simulink model "battery_sim"  (R2022a)
settings: Solver=VariableStepAuto  StartTime=0.0  StopTime=10000  RelTol=1e-3
undefined symbols (not defined in the file): T_AMB
settings Model: Creator=Cristobal  LastModifiedBy=Cristobal

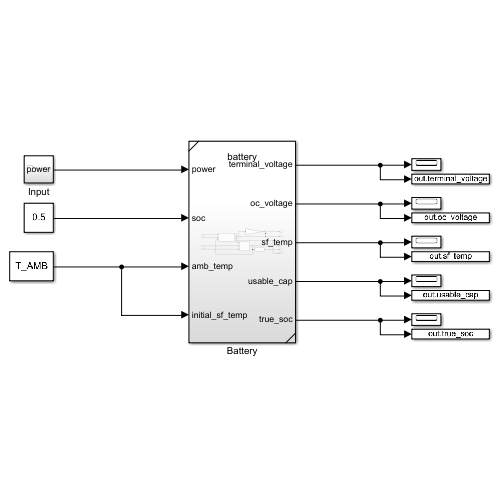
[thumbnail: Simulink's stored preview of the top-level diagram]
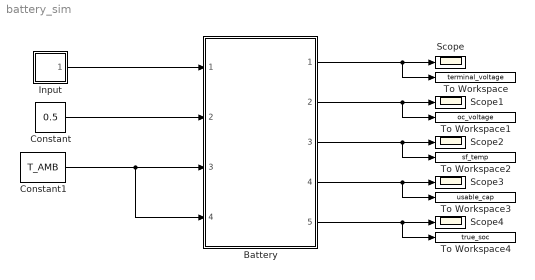
== system battery_sim ==
  Battery : Subsystem  ReferencedSubsystem=battery
  Constant : Constant  Value=0.5
  Constant1 : Constant  Value=T_AMB
  Input : Subsystem
  Scope{,1..4} (5 alike) : Scope
  To Workspace : ToWorkspace  VariableName=terminal_voltage  SaveFormat=Timeseries  SampleTime=-1
  To Workspace1 : ToWorkspace  VariableName=oc_voltage  SaveFormat=Timeseries  SampleTime=-1
  To Workspace2 : ToWorkspace  VariableName=sf_temp  SaveFormat=Timeseries  SampleTime=-1
  To Workspace3 : ToWorkspace  VariableName=usable_cap  SaveFormat=Timeseries  SampleTime=-1
  To Workspace4 : ToWorkspace  VariableName=true_soc  SaveFormat=Timeseries  SampleTime=-1
  wires:
  Input/1(power) -> Battery/1
  Constant/1 -> Battery/2
  Constant1/1 -> Battery/4, Battery/3
  Battery/1 -> Scope/1, To Workspace/1
  Battery/2 -> Scope1/1, To Workspace1/1
  Battery/3 -> Scope2/1, To Workspace2/1
  Battery/4 -> Scope3/1, To Workspace3/1
  Battery/5 -> Scope4/1, To Workspace4/1

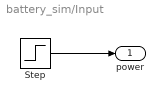
== system battery_sim/Input ==
  Step : Step  After=100  SampleTime=0
  power : Outport
  wires:
  Step/1 -> power/1
